simulink model "stereo_ibvs_core_backup_20260724_032606"  (R2025b)
settings: Solver=FixedStepDiscrete  StartTime=0.0  StopTime=10  FixedStep=cfg.Ts  RelTol=1e-3
InitFcn:
  | modelPath = get_param(bdroot,'FileName');
  |                                                                                       simulinkPath = fileparts(fileparts(modelPath));
  |                                                                                       configPath = fullfile(simulinkPath,'config','stereo_ibvs_config.m');
  |                                                                                       if ~isfile(configPath), error('StereoIBVS:ConfigNotFound','找不到配置文件：%s',configPath); end
  |                                                                                       run(configPath);
undefined symbols (not defined in the file): cfg
(part 4 of 4)

== matlab function stereo_ibvs_core_backup_20260724_032606/09_Safety_Supervisor/Apply Safety and Saturation ==
  data: qDotCmd input; qDotApplied output; fDotMmLimited input; q input; focalLengthMeasuredMm input; validLeft input; focalLengthFresh input; cameraModelValid input; kinematicsValid input; JL input; controllerEnableSafe input; cfg_qDotMax input; cfg_qDotAlgorithmMax input; cfg_qMin input; cfg_qMax input; cfg_qLimitSoftMargin input; cfg_cartesianLinearSpeedMax input; cfg_focalRateGuaranteedMmPerSec input; cfg_focalRateAbsoluteMaxMmPerSec input; cfg_focalLengthWorkingMinMm input; cfg_focalLengthWorkingMaxMm input; cfg_focalLengthHardwareMinMm input; cfg_focalLengthHardwareMaxMm input; cfg_Ts input; cfg_numericalEpsilon input; cfg_armControlCalibrationReady input; cfg_zoomControlCalibrationReady input; cfg_armControlEnable input; cfg_zoomControlEnable input; fDotMmApplied output; qSaturationFlag output; focalRateSaturationFlag output; jointVelocitySaturationFlag output; jointVelocitySaturationAny output; jointLimitWarning output; cartesianSpeed output; cartesianSpeedScale output; cartesianSpeedSaturationFlag output; focalLengthCommandMm output; focalRateUsageGuaranteed output; focalRateUsageHard output; focalRateHardViolation output; safetyValid output
function [ ...
    qDotApplied, ...
    fDotMmApplied, ...
    qSaturationFlag, ...
    focalRateSaturationFlag, ...
    jointVelocitySaturationFlag, ...
    jointVelocitySaturationAny, ...
    jointLimitWarning, ...
    cartesianSpeed, ...
    cartesianSpeedScale, ...
    cartesianSpeedSaturationFlag, ...
    focalLengthCommandMm, ...
    focalRateUsageGuaranteed, ...
    focalRateUsageHard, ...
    focalRateHardViolation, ...
    safetyValid] = fcn( ...
    qDotCmd, ...
    fDotMmLimited, ...
    q, ...
    focalLengthMeasuredMm, ...
    validLeft, ...
    focalLengthFresh, ...
    cameraModelValid, ...
    kinematicsValid, ...
    JL, ...
    controllerEnableSafe, ...
    cfg_qDotMax, ...
    cfg_qDotAlgorithmMax, ...
    cfg_qMin, ...
    cfg_qMax, ...
    cfg_qLimitSoftMargin, ...
    cfg_cartesianLinearSpeedMax, ...
    cfg_focalRateGuaranteedMmPerSec, ...
    cfg_focalRateAbsoluteMaxMmPerSec, ...
    cfg_focalLengthWorkingMinMm, ...
    cfg_focalLengthWorkingMaxMm, ...
    cfg_focalLengthHardwareMinMm, ...
    cfg_focalLengthHardwareMaxMm, ...
    cfg_Ts, ...
    cfg_numericalEpsilon, ...
    cfg_armControlCalibrationReady, ...
    cfg_zoomControlCalibrationReady, ...
    cfg_armControlEnable, ...
    cfg_zoomControlEnable)
%#codegen
% V2 Safety and Saturation
% JL顺序：[linear velocity; angular velocity]

%% 固定尺寸输出
qDotApplied = zeros(7,1);
fDotMmApplied = zeros(2,1);

qSaturationFlag = 0;
focalRateSaturationFlag = 0;

jointVelocitySaturationFlag = zeros(7,1);
jointVelocitySaturationAny = 0;
jointLimitWarning = zeros(7,1);

cartesianSpeed = 0;
cartesianSpeedScale = 1;
cartesianSpeedSaturationFlag = 0;

focalLengthCommandMm = zeros(2,1);
focalRateUsageGuaranteed = zeros(2,1);
focalRateUsageHard = zeros(2,1);
focalRateHardViolation = zeros(2,1);

safetyValid = 0;

%% 固定尺寸输入
qDotRequested = reshape(qDotCmd,7,1);
fDotRequested = reshape(fDotMmLimited,2,1);
qMeasured = reshape(q,7,1);
focalMeasured = reshape(focalLengthMeasuredMm,2,1);

%% 参数检查
tol = max(cfg_numericalEpsilon,1e-12);

inputFinite = ...
    all(isfinite(qDotRequested)) && ...
    all(isfinite(fDotRequested)) && ...
    all(isfinite(qMeasured)) && ...
    all(isfinite(focalMeasured)) && ...
    all(isfinite(JL(:))) && ...
    isfinite(validLeft) && ...
    isfinite(focalLengthFresh) && ...
    isfinite(cameraModelValid) && ...
    isfinite(kinematicsValid) && ...
    isfinite(controllerEnableSafe);

parameterFinite = ...
    all(isfinite(cfg_qDotMax)) && ...
    all(isfinite(cfg_qDotAlgorithmMax)) && ...
    all(isfinite(cfg_qMin)) && ...
    all(isfinite(cfg_qMax)) && ...
    isfinite(cfg_qLimitSoftMargin) && ...
    isfinite(cfg_cartesianLinearSpeedMax) && ...
    isfinite(cfg_focalRateGuaranteedMmPerSec) && ...
    isfinite(cfg_focalRateAbsoluteMaxMmPerSec) && ...
    all(isfinite(cfg_focalLengthWorkingMinMm)) && ...
    all(isfinite(cfg_focalLengthWorkingMaxMm)) && ...
    all(isfinite(cfg_focalLengthHardwareMinMm)) && ...
    all(isfinite(cfg_focalLengthHardwareMaxMm)) && ...
    isfinite(cfg_Ts) && ...
    isfinite(cfg_numericalEpsilon) && ...
    isfinite(cfg_armControlCalibrationReady) && ...
    isfinite(cfg_zoomControlCalibrationReady) && ...
    isfinite(cfg_armControlEnable) && ...
    isfinite(cfg_zoomControlEnable);

parameterRangesValid = ...
    all(cfg_qDotMax >= 0) && ...
    all(cfg_qDotAlgorithmMax >= 0) && ...
    all(cfg_qMax > cfg_qMin) && ...
    cfg_qLimitSoftMargin >= 0 && ...
    all(2*cfg_qLimitSoftMargin < ...
        (cfg_qMax-cfg_qMin)) && ...
    cfg_cartesianLinearSpeedMax > 0 && ...
    cfg_focalRateGuaranteedMmPerSec > 0 && ...
    cfg_focalRateAbsoluteMaxMmPerSec >= ...
        cfg_focalRateGuaranteedMmPerSec && ...
    all(cfg_focalLengthHardwareMaxMm > ...
        cfg_focalLengthHardwareMinMm) && ...
    all(cfg_focalLengthWorkingMinMm >= ...
        cfg_focalLengthHardwareMinMm) && ...
    all(cfg_focalLengthWorkingMaxMm <= ...
        cfg_focalLengthHardwareMaxMm) && ...
    all(cfg_focalLengthWorkingMaxMm > ...
        cfg_focalLengthWorkingMinMm) && ...
    cfg_Ts > 0;

if ~(inputFinite && parameterFinite && parameterRangesValid)
    qSaturationFlag = 1;
    focalRateSaturationFlag = 1;
    jointVelocitySaturationFlag = ones(7,1);
    jointVelocitySaturationAny = 1;
    cartesianSpeedScale = 0;
    return;
end

safetyValid = 1;

%% 当前焦距
if cameraModelValid > 0.5
    focalLengthCommandMm = focalMeasured;
end

%% 关节限位诊断
for i = 1:7
    nearLowerLimit = ...
        qMeasured(i) <= ...
        cfg_qMin(i)+cfg_qLimitSoftMargin;

    nearUpperLimit = ...
        qMeasured(i) >= ...
        cfg_qMax(i)-cfg_qLimitSoftMargin;

    outsideLowerLimit = ...
        qMeasured(i) <= cfg_qMin(i);

    outsideUpperLimit = ...
        qMeasured(i) >= cfg_qMax(i);

    jointLimitWarning(i) = double( ...
        nearLowerLimit || ...
        nearUpperLimit || ...
        outsideLowerLimit || ...
        outsideUpperLimit);
end

%% 控制许可
armPermission = ...
    controllerEnableSafe > 0.5 && ...
    cfg_armControlEnable > 0.5 && ...
    cfg_armControlCalibrationReady > 0.5 && ...
    validLeft > 0.5 && ...
    cameraModelValid > 0.5 && ...
    kinematicsValid > 0.5;

zoomPermission = ...
    controllerEnableSafe > 0.5 && ...
    cfg_zoomControlEnable > 0.5 && ...
    cfg_zoomControlCalibrationReady > 0.5 && ...
    validLeft > 0.5 && ...
    cameraModelValid > 0.5 && ...
    focalLengthFresh > 0.5;

%% 关节速度整组同比例限制
if armPermission

    qDotLimit = min( ...
        abs(cfg_qDotMax), ...
        abs(cfg_qDotAlgorithmMax));

    qDotRatio = ...
        abs(qDotRequested) ./ ...
        max(qDotLimit,tol);

    qDotScale = max(1,max(qDotRatio));
    qCandidate = qDotRequested/qDotScale;

    for i = 1:7

        nearLowerLimit = ...
            qMeasured(i) <= ...
            cfg_qMin(i)+cfg_qLimitSoftMargin;

        nearUpperLimit = ...
            qMeasured(i) >= ...
            cfg_qMax(i)-cfg_qLimitSoftMargin;

        if nearLowerLimit && qCandidate(i) < 0
            qCandidate(i) = 0;
        end

        if nearUpperLimit && qCandidate(i) > 0
            qCandidate(i) = 0;
        end
    end

    %% 笛卡尔线速度限制
    cameraTwistCandidate = JL*qCandidate;
    cartesianSpeedCandidate = ...
        norm(cameraTwistCandidate(1:3));

    if ~isfinite(cartesianSpeedCandidate)

        qCandidate = zeros(7,1);
        cartesianSpeedScale = 0;
        cartesianSpeedSaturationFlag = 1;
        safetyValid = 0;

    elseif cartesianSpeedCandidate > ...
            cfg_cartesianLinearSpeedMax

        cartesianSpeedScale = ...
            cfg_cartesianLinearSpeedMax / ...
            max(cartesianSpeedCandidate,tol);

        qCandidate = ...
            cartesianSpeedScale*qCandidate;

        cartesianSpeedSaturationFlag = 1;
    end

    qDotApplied = min( ...
        max(qCandidate,-qDotLimit), ...
        qDotLimit);

    finalCameraTwist = JL*qDotApplied;
    cartesianSpeed = norm(finalCameraTwist(1:3));
end

%% Zoom硬限速违规诊断
focalRateHardViolation = double( ...
    abs(fDotRequested) > ...
    cfg_focalRateAbsoluteMaxMmPerSec);

%% Zoom焦距速度限制
if zoomPermission

    fCandidate = min( ...
        max(fDotRequested, ...
            -cfg_focalRateAbsoluteMaxMmPerSec), ...
        cfg_focalRateAbsoluteMaxMmPerSec);

    for i = 1:2

        focalCurrent = focalMeasured(i);

        workingMin = ...
            cfg_focalLengthWorkingMinMm(i);
        workingMax = ...
            cfg_focalLengthWorkingMaxMm(i);

        hardwareMin = ...
            cfg_focalLengthHardwareMinMm(i);
        hardwareMax = ...
            cfg_focalLengthHardwareMaxMm(i);

        %% 禁止继续远离工作范围
        if focalCurrent <= workingMin && ...
                fCandidate(i) < 0
            fCandidate(i) = 0;
        end

        if focalCurrent >= workingMax && ...
                fCandidate(i) > 0
            fCandidate(i) = 0;
        end

        %% 下一周期工作范围预测
        nextFocalLength = ...
            focalCurrent + ...
            cfg_Ts*fCandidate(i);

        if focalCurrent >= workingMin && ...
                nextFocalLength < workingMin

            fCandidate(i) = ...
                (workingMin-focalCurrent)/cfg_Ts;

        elseif focalCurrent <= workingMax && ...
                nextFocalLength > workingMax

            fCandidate(i) = ...
                (workingMax-focalCurrent)/cfg_Ts;
        end

        %% 硬件范围最终保护
        nextFocalLength = ...
            focalCurrent + ...
            cfg_Ts*fCandidate(i);

        if nextFocalLength < hardwareMin

            fCandidate(i) = ...
                (hardwareMin-focalCurrent)/cfg_Ts;

        elseif nextFocalLength > hardwareMax

            fCandidate(i) = ...
                (hardwareMax-focalCurrent)/cfg_Ts;
        end
    end

    fDotMmApplied = min( ...
        max(fCandidate, ...
            -cfg_focalRateAbsoluteMaxMmPerSec), ...
        cfg_focalRateAbsoluteMaxMmPerSec);
end

%% 最终有限值保护
if any(~isfinite(qDotApplied)) || ...
        ~isfinite(cartesianSpeed) || ...
        ~isfinite(cartesianSpeedScale)

    qDotApplied = zeros(7,1);
    cartesianSpeed = 0;
    cartesianSpeedScale = 0;
    cartesianSpeedSaturationFlag = 1;
    safetyValid = 0;
end

if any(~isfinite(fDotMmApplied))
    fDotMmApplied = zeros(2,1);
    safetyValid = 0;
end

%% 饱和诊断
jointVelocitySaturationFlag = double( ...
    abs(qDotApplied-qDotRequested) > tol);

jointVelocitySaturationAny = double( ...
    any(jointVelocitySaturationFlag > 0.5));

qSaturationFlag = ...
    jointVelocitySaturationAny;

focalRateSaturationFlag = double( ...
    any(abs(fDotMmApplied-fDotRequested) > tol));

%% Zoom使用率
focalRateUsageGuaranteed = ...
    abs(fDotMmApplied) / ...
    cfg_focalRateGuaranteedMmPerSec;

focalRateUsageHard = ...
    abs(fDotMmApplied) / ...
    cfg_focalRateAbsoluteMaxMmPerSec;

%% 下一周期焦距命令
if cameraModelValid > 0.5

    focalLengthCommandMm = min( ...
        max( ...
            focalMeasured + ...
            cfg_Ts*fDotMmApplied, ...
            cfg_focalLengthHardwareMinMm), ...
        cfg_focalLengthHardwareMaxMm);

else
    focalLengthCommandMm = zeros(2,1);
end

%% 最终输出检查
if any(~isfinite(focalLengthCommandMm)) || ...
        any(~isfinite(focalRateUsageGuaranteed)) || ...
        any(~isfinite(focalRateUsageHard))

    fDotMmApplied = zeros(2,1);
    focalLengthCommandMm = zeros(2,1);
    focalRateUsageGuaranteed = zeros(2,1);
    focalRateUsageHard = zeros(2,1);
    safetyValid = 0;
end
end

== matlab function stereo_ibvs_core_backup_20260724_032606/10_Diagnostics/V2_Output_and_Diagnostics ==
  data: qDotApplied input; jointVelocityCmd output; fDotMmApplied input; inputDataValid input; cameraModelValid input; focalLengthFresh input; kinematicsValid input; validLeft input; validRight input; validStereoQualified input; ekfPredictionValid input; ekfMeasurementUpdated input; depthTaskWeight input; schedulerMode input; safetyValid input; controllerEnableSafe input; focalRateCmdMmPerSec output; controllerStatus output
function [ ...
    jointVelocityCmd, ...
    focalRateCmdMmPerSec, ...
    controllerStatus] = fcn( ...
    qDotApplied, ...
    fDotMmApplied, ...
    inputDataValid, ...
    cameraModelValid, ...
    focalLengthFresh, ...
    kinematicsValid, ...
    validLeft, ...
    validRight, ...
    validStereoQualified, ...
    ekfPredictionValid, ...
    ekfMeasurementUpdated, ...
    depthTaskWeight, ...
    schedulerMode, ...
    safetyValid, ...
    controllerEnableSafe)
%#codegen
% V2 Output and Diagnostics
%
% jointVelocityCmd:
% [qDot1; ...; qDot7]，单位 rad/s
%
% focalRateCmdMmPerSec:
% [fDotLeft; fDotRight]，单位 mm/s
%
% 不再进行焦距速度到step/s的转换。

%% 固定尺寸输出
jointVelocityCmd = zeros(7,1);
focalRateCmdMmPerSec = zeros(2,1);
controllerStatus = zeros(13,1);

%% 固定尺寸输入
qDot = reshape(qDotApplied,7,1);
fDotMm = reshape(fDotMmApplied,2,1);

%% 状态信号整理
statusInputDataValid = double( ...
    isfinite(inputDataValid) && ...
    inputDataValid > 0.5);

statusCameraModelValid = double( ...
    isfinite(cameraModelValid) && ...
    cameraModelValid > 0.5);

statusFocalLengthFresh = double( ...
    isfinite(focalLengthFresh) && ...
    focalLengthFresh > 0.5);

statusKinematicsValid = double( ...
    isfinite(kinematicsValid) && ...
    kinematicsValid > 0.5);

statusValidLeft = double( ...
    isfinite(validLeft) && ...
    validLeft > 0.5);

statusValidRight = double( ...
    isfinite(validRight) && ...
    validRight > 0.5);

statusValidStereoQualified = double( ...
    isfinite(validStereoQualified) && ...
    validStereoQualified > 0.5);

statusEkfPredictionValid = double( ...
    isfinite(ekfPredictionValid) && ...
    ekfPredictionValid > 0.5);

statusEkfMeasurementUpdated = double( ...
    isfinite(ekfMeasurementUpdated) && ...
    ekfMeasurementUpdated > 0.5);

if isfinite(depthTaskWeight)
    statusDepthTaskWeight = ...
        min(max(depthTaskWeight,0),1);
else
    statusDepthTaskWeight = 0;
end

if isfinite(schedulerMode)
    statusSchedulerMode = schedulerMode;
else
    statusSchedulerMode = 0;
end

statusSafetyValid = double( ...
    isfinite(safetyValid) && ...
    safetyValid > 0.5);

statusControllerEnableSafe = double( ...
    isfinite(controllerEnableSafe) && ...
    controllerEnableSafe > 0.5);

%% 固定顺序状态数组
controllerStatus = [
    statusInputDataValid
    statusCameraModelValid
    statusFocalLengthFresh
    statusKinematicsValid
    statusValidLeft
    statusValidRight
    statusValidStereoQualified
    statusEkfPredictionValid
    statusEkfMeasurementUpdated
    statusDepthTaskWeight
    statusSchedulerMode
    statusSafetyValid
    statusControllerEnableSafe
];

%% 最终机械臂输出许可
armCommandEnable = ...
    all(isfinite(qDot)) && ...
    statusInputDataValid > 0.5 && ...
    statusCameraModelValid > 0.5 && ...
    statusKinematicsValid > 0.5 && ...
    statusValidLeft > 0.5 && ...
    statusSafetyValid > 0.5 && ...
    statusControllerEnableSafe > 0.5;

if armCommandEnable
    jointVelocityCmd = qDot;
end

%% 最终Zoom输出许可
zoomCommandEnable = ...
    all(isfinite(fDotMm)) && ...
    statusInputDataValid > 0.5 && ...
    statusCameraModelValid > 0.5 && ...
    statusFocalLengthFresh > 0.5 && ...
    statusValidLeft > 0.5 && ...
    statusSafetyValid > 0.5 && ...
    statusControllerEnableSafe > 0.5;

if zoomCommandEnable
    focalRateCmdMmPerSec = fDotMm;
end

%% 最终有限值保护
if any(~isfinite(jointVelocityCmd))
    jointVelocityCmd = zeros(7,1);
end

if any(~isfinite(focalRateCmdMmPerSec))
    focalRateCmdMmPerSec = zeros(2,1);
end

if any(~isfinite(controllerStatus))
    controllerStatus = zeros(13,1);
end
end

== matlab function stereo_ibvs_core_backup_20260724_032606/Split Vision Feature ==
  data: visionFeature input; validLeft output; validRight output; pixelMeasurement output; scaleMeasuredRaw output
function [validLeft,validRight,pixelMeasurement,scaleMeasuredRaw] = fcn(visionFeature)
%#codegen
feature = reshape(visionFeature,8,1);
validLeft = feature(1);
validRight = feature(2);
pixelMeasurement = feature(3:6);
scaleMeasuredRaw = feature(7:8);
end

== matlab function stereo_ibvs_core_backup_20260724_032606/Target Velocity Frame Transform ==
  data: vHatW input; vHatCR output; RWCR input
function vHatCR = fcn(vHatW,RWCR)
%#codegen
vHatCR = zeros(3,1);
velocityW = reshape(vHatW,3,1);
rotationCRToW = reshape(RWCR,3,3);
if all(isfinite(velocityW)) && all(isfinite(rotationCRToW(:)))
    vHatCR = rotationCRToW'*velocityW;
end
end

== matlab function stereo_ibvs_core_backup_20260724_032606/02_Camera_and_Zoom_Model/V2_Camera_and_Zoom_Model ==
  data: focalLengthMeasuredMmRaw input; focalLengthMeasuredMm output; focalLengthIsNew input; resetSafe input; cfg_focalLengthHardwareMinMm input; cfg_focalLengthHardwareMaxMm input; cfg_focalLengthWorkingMinMm input; cfg_focalLengthWorkingMaxMm input; cfg_outputPixelPitchXmm input; cfg_outputPixelPitchYmm input; cfg_focalLengthTimeoutFrames input; cfg_numericalEpsilon input; fxMeasuredPx output; fyMeasuredPx output; focalLengthFresh output; focalLengthDataValid output; focalAtWorkingLowerLimit output; focalAtWorkingUpperLimit output; focalAtHardwareLowerLimit output; focalAtHardwareUpperLimit output; focalOutsideWorkingRange output; focalHardwareLimitViolation output; focalRangeUsage output; focalHeadroomMm output; cameraModelValid output
function [ ...
    focalLengthMeasuredMm, ...
    fxMeasuredPx, ...
    fyMeasuredPx, ...
    focalLengthFresh, ...
    focalLengthDataValid, ...
    focalAtWorkingLowerLimit, ...
    focalAtWorkingUpperLimit, ...
    focalAtHardwareLowerLimit, ...
    focalAtHardwareUpperLimit, ...
    focalOutsideWorkingRange, ...
    focalHardwareLimitViolation, ...
    focalRangeUsage, ...
    focalHeadroomMm, ...
    cameraModelValid] = fcn( ...
    focalLengthMeasuredMmRaw, ...
    focalLengthIsNew, ...
    resetSafe, ...
    cfg_focalLengthHardwareMinMm, ...
    cfg_focalLengthHardwareMaxMm, ...
    cfg_focalLengthWorkingMinMm, ...
    cfg_focalLengthWorkingMaxMm, ...
    cfg_outputPixelPitchXmm, ...
    cfg_outputPixelPitchYmm, ...
    cfg_focalLengthTimeoutFrames, ...
    cfg_numericalEpsilon)
%#codegen
% V2 Camera and Zoom Model
%
% 焦距反馈：
% [fL_mm; fR_mm]
%
% 超时后保持最后一次有效焦距，但 focalLengthFresh = false。
% 08模块应在 focalLengthFresh = false 时停止Zoom命令。

%% 固定尺寸输入
focalRaw = reshape(focalLengthMeasuredMmRaw,2,1);

hardwareMin = reshape( ...
    cfg_focalLengthHardwareMinMm,2,1);

hardwareMax = reshape( ...
    cfg_focalLengthHardwareMaxMm,2,1);

workingMin = reshape( ...
    cfg_focalLengthWorkingMinMm,2,1);

workingMax = reshape( ...
    cfg_focalLengthWorkingMaxMm,2,1);

%% 持久状态
persistent lastValidFocalLengthMm
persistent focalLengthReceivedOnce
persistent framesSinceLastValidMessage

if isempty(lastValidFocalLengthMm)
    lastValidFocalLengthMm = zeros(2,1);
    focalLengthReceivedOnce = false;
    framesSinceLastValidMessage = ...
        double(cfg_focalLengthTimeoutFrames);
end

%% 固定尺寸输出
focalLengthMeasuredMm = zeros(2,1);
fxMeasuredPx = zeros(2,1);
fyMeasuredPx = zeros(2,1);

focalLengthFresh = 0;
focalLengthDataValid = 0;
focalAtWorkingLowerLimit = zeros(2,1);
focalAtWorkingUpperLimit = zeros(2,1);
focalAtHardwareLowerLimit = zeros(2,1);
focalAtHardwareUpperLimit = zeros(2,1);
focalOutsideWorkingRange = zeros(2,1);
focalHardwareLimitViolation = zeros(2,1);

focalRangeUsage = zeros(2,1);
focalHeadroomMm = zeros(2,1);

cameraModelValid = 0;

%% 配置检查
numericalConfigurationValid = ...
    isfinite(cfg_numericalEpsilon) && ...
    cfg_numericalEpsilon > 0;

hardwareRangeValid = ...
    all(isfinite(hardwareMin)) && ...
    all(isfinite(hardwareMax)) && ...
    all(hardwareMax > hardwareMin);

workingRangeValid = ...
    all(isfinite(workingMin)) && ...
    all(isfinite(workingMax)) && ...
    all(workingMax > workingMin) && ...
    all(workingMin >= hardwareMin) && ...
    all(workingMax <= hardwareMax);

pixelPitchValid = ...
    isfinite(cfg_outputPixelPitchXmm) && ...
    isfinite(cfg_outputPixelPitchYmm) && ...
    cfg_outputPixelPitchXmm > cfg_numericalEpsilon && ...
    cfg_outputPixelPitchYmm > cfg_numericalEpsilon;

timeoutConfigurationValid = ...
    isfinite(cfg_focalLengthTimeoutFrames) && ...
    cfg_focalLengthTimeoutFrames >= 1;

configurationValid = ...
    numericalConfigurationValid && ...
    hardwareRangeValid && ...
    workingRangeValid && ...
    pixelPitchValid && ...
    timeoutConfigurationValid;

%% 控制输入检查
controlSignalsFinite = ...
    isfinite(focalLengthIsNew) && ...
    isfinite(resetSafe);

%% 复位或更新焦距状态
if ~controlSignalsFinite || resetSafe > 0.5

    lastValidFocalLengthMm = zeros(2,1);
    focalLengthReceivedOnce = false;
    framesSinceLastValidMessage = ...
        double(cfg_focalLengthTimeoutFrames);

else

    rawFinite = all(isfinite(focalRaw));

    rawInsideHardwareRange = ...
        rawFinite && ...
        hardwareRangeValid && ...
        all(focalRaw >= hardwareMin) && ...
        all(focalRaw <= hardwareMax);

    newValidMessage = ...
        focalLengthIsNew > 0.5 && ...
        rawInsideHardwareRange && ...
        configurationValid;

    if newValidMessage

        lastValidFocalLengthMm = focalRaw;
        focalLengthReceivedOnce = true;
        framesSinceLastValidMessage = 0;

    elseif focalLengthReceivedOnce

        maximumCounterValue = ...
            double(cfg_focalLengthTimeoutFrames) + 1;

        framesSinceLastValidMessage = min( ...
            framesSinceLastValidMessage + 1, ...
            maximumCounterValue);
    end
end

%% 输出最近一次有效焦距
if focalLengthReceivedOnce
    focalLengthMeasuredMm = ...
        lastValidFocalLengthMm;
end

%% 焦距新鲜度
focalLengthFresh = double( ...
    focalLengthReceivedOnce && ...
    framesSinceLastValidMessage < ...
        double(cfg_focalLengthTimeoutFrames));

%% 保存焦距有效性
if focalLengthReceivedOnce && hardwareRangeValid

    focalLengthDataValid = double( ...
        all(isfinite(focalLengthMeasuredMm)) && ...
        all(focalLengthMeasuredMm >= hardwareMin) && ...
        all(focalLengthMeasuredMm <= hardwareMax));
end

%% 焦距范围状态
if focalLengthReceivedOnce && configurationValid

    focalAtWorkingLowerLimit = double( ...
        focalLengthMeasuredMm <= workingMin);

    focalAtWorkingUpperLimit = double( ...
        focalLengthMeasuredMm >= workingMax);

    focalAtHardwareLowerLimit = double( ...
        focalLengthMeasuredMm <= hardwareMin);

    focalAtHardwareUpperLimit = double( ...
        focalLengthMeasuredMm >= hardwareMax);

    focalOutsideWorkingRange = double( ...
        focalLengthMeasuredMm < workingMin | ...
        focalLengthMeasuredMm > workingMax);

    focalHardwareLimitViolation = double( ...
        focalLengthMeasuredMm < hardwareMin | ...
        focalLengthMeasuredMm > hardwareMax);

    workingRangeWidth = ...
        workingMax - workingMin;

    focalRangeUsage = ...
        (focalLengthMeasuredMm-workingMin) ./ ...
        workingRangeWidth;

    focalRangeUsage = min( ...
        max(focalRangeUsage,zeros(2,1)), ...
        ones(2,1));

    lowerHeadroomMm = ...
        focalLengthMeasuredMm-workingMin;

    upperHeadroomMm = ...
        workingMax-focalLengthMeasuredMm;

    focalHeadroomMm = max( ...
        min(lowerHeadroomMm,upperHeadroomMm), ...
        zeros(2,1));
end

%% 焦距mm转换为像素焦距
cameraModelValid = double( ...
    configurationValid && ...
    focalLengthDataValid > 0.5 && ...
    ~any(focalHardwareLimitViolation > 0.5));

if cameraModelValid

    fxMeasuredPx = ...
        focalLengthMeasuredMm ./ ...
        cfg_outputPixelPitchXmm;

    fyMeasuredPx = ...
        focalLengthMeasuredMm ./ ...
        cfg_outputPixelPitchYmm;
end

%% 最终有限值保护
outputFinite = ...
    all(isfinite(focalLengthMeasuredMm)) && ...
    all(isfinite(fxMeasuredPx)) && ...
    all(isfinite(fyMeasuredPx)) && ...
    all(isfinite(focalRangeUsage)) && ...
    all(isfinite(focalHeadroomMm));

if ~outputFinite

    focalLengthMeasuredMm = zeros(2,1);
    fxMeasuredPx = zeros(2,1);
    fyMeasuredPx = zeros(2,1);

    focalLengthFresh = 0;
    focalLengthDataValid = 0;

    focalAtWorkingLowerLimit = zeros(2,1);
    focalAtWorkingUpperLimit = zeros(2,1);
    focalAtHardwareLowerLimit = zeros(2,1);
    focalAtHardwareUpperLimit = zeros(2,1);

    focalOutsideWorkingRange = zeros(2,1);
    focalHardwareLimitViolation = zeros(2,1);

    focalRangeUsage = zeros(2,1);
    focalHeadroomMm = zeros(2,1);

    cameraModelValid = 0;
end
end

== matlab function stereo_ibvs_core_backup_20260724_032606/01_Input_Validity/Input Validity ==
  data: qRaw input; q output; visionFeatureRaw input; focalLengthMeasuredMmRaw input; visionMeasurementNewRaw input; focalLengthIsNewRaw input; controllerEnableRaw input; resetRaw input; qInitial input; focalLength0Mm input; visionTimeoutFrames input; visionFeature output; focalLengthMeasuredMm output; visionMeasurementNewSafe output; focalLengthIsNewSafe output; controllerEnableSafe output; resetSafe output; inputDataValid output
function [ ...
    q, ...
    visionFeature, ...
    focalLengthMeasuredMm, ...
    visionMeasurementNewSafe, ...
    focalLengthIsNewSafe, ...
    controllerEnableSafe, ...
    resetSafe, ...
    inputDataValid] = fcn( ...
    qRaw, ...
    visionFeatureRaw, ...
    focalLengthMeasuredMmRaw, ...
    visionMeasurementNewRaw, ...
    focalLengthIsNewRaw, ...
    controllerEnableRaw, ...
    resetRaw, ...
    qInitial, ...
    focalLength0Mm, ...
    visionTimeoutFrames)
%#codegen
% 检查并保存最近一次合法的关节、视觉和焦距输入。
% Core内部焦距统一使用mm。
% 视觉消息超时后inputDataValid和controllerEnableSafe立即归零。

persistent lastQ
persistent lastVisionFeature
persistent lastFocalLengthMeasuredMm
persistent visionReceivedOnce
persistent framesSinceLastVisionMessage

initialQ = reshape(qInitial,7,1);
initialFocalLengthMm = reshape(focalLength0Mm,2,1);

timeoutConfigurationValid = ...
    isfinite(visionTimeoutFrames) && ...
    visionTimeoutFrames >= 1;

timeoutFrames = 1.0;
if timeoutConfigurationValid
    timeoutFrames = max(1.0,floor(visionTimeoutFrames));
end

if isempty(lastQ)
    lastQ = initialQ;
    lastVisionFeature = zeros(8,1);
    lastFocalLengthMeasuredMm = initialFocalLengthMm;
    visionReceivedOnce = false;
    framesSinceLastVisionMessage = timeoutFrames;
end

qCandidate = reshape(qRaw,7,1);
visionCandidate = reshape(visionFeatureRaw,8,1);
focalCandidate = reshape(focalLengthMeasuredMmRaw,2,1);

qValid = all(isfinite(qCandidate));
visionValid = all(isfinite(visionCandidate));
focalValid = all(isfinite(focalCandidate));
visionNewValid = isfinite(visionMeasurementNewRaw);
focalNewValid = isfinite(focalLengthIsNewRaw);
enableValid = isfinite(controllerEnableRaw);
resetValid = isfinite(resetRaw);

newVisionMessage = ...
    visionNewValid && ...
    visionMeasurementNewRaw > 0.5;

newFocalMessage = ...
    focalNewValid && ...
    focalLengthIsNewRaw > 0.5;

visionMeasurementNewSafe = double( ...
    newVisionMessage && visionValid);

focalLengthIsNewSafe = double( ...
    newFocalMessage && focalValid);

if qValid
    lastQ = qCandidate;
end

if visionMeasurementNewSafe > 0.5
    lastVisionFeature = visionCandidate;
    visionReceivedOnce = true;
    framesSinceLastVisionMessage = 0;
elseif visionReceivedOnce
    framesSinceLastVisionMessage = min( ...
        framesSinceLastVisionMessage + 1, ...
        timeoutFrames + 1);
end

if focalLengthIsNewSafe > 0.5
    lastFocalLengthMeasuredMm = focalCandidate;
end

q = lastQ;
visionFeature = lastVisionFeature;
focalLengthMeasuredMm = lastFocalLengthMeasuredMm;

visionFresh = ...
    visionReceivedOnce && ...
    framesSinceLastVisionMessage < timeoutFrames;

inputDataValid = double( ...
    qValid && ...
    focalValid && ...
    visionNewValid && ...
    focalNewValid && ...
    enableValid && ...
    resetValid && ...
    timeoutConfigurationValid && ...
    visionFresh);

controllerEnableSafe = double( ...
    inputDataValid > 0.5 && ...
    controllerEnableRaw > 0.5);

if resetValid
    resetSafe = double(resetRaw > 0.5);
else
    resetSafe = 0;
end

if resetSafe > 0.5
    lastQ = initialQ;
    lastVisionFeature = zeros(8,1);
    lastFocalLengthMeasuredMm = initialFocalLengthMm;
    visionReceivedOnce = false;
    framesSinceLastVisionMessage = timeoutFrames;

    q = lastQ;
    visionFeature = lastVisionFeature;
    focalLengthMeasuredMm = lastFocalLengthMeasuredMm;
    visionMeasurementNewSafe = 0;
    focalLengthIsNewSafe = 0;
    controllerEnableSafe = 0;
    inputDataValid = 0;
end
end
